simulink model "untitled_H"  (R2013b)
settings: Solver=ode45  StartTime=0.0  StopTime=500  RelTol=1e-3
undefined symbols (not defined in the file): c, delta, kappa, kd, ki, kp, Qs
libraries: simulink x1
settings Model: Creator=Yurii  LastModifiedBy=Yurii

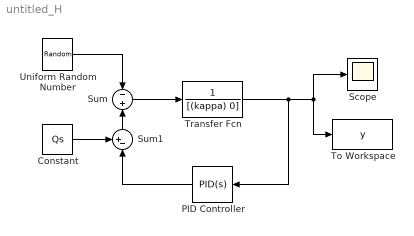
== system untitled_H ==
  Constant : Constant  Value=Qs
  PID Controller : simulink/Continuous/PID Controller  Controller=PID  TimeDomain=Continuous-time  SampleTime=1  IntegratorMethod=Forward Euler  FilterMethod=Forward Euler  Form=Parallel  P=kp  I=ki  D=kd  N=100  InitialConditionSource=internal  InitialConditionForIntegrator=0  InitialConditionForFilter=0  ExternalReset=none  LimitOutput=off  UpperSaturationLimit=inf  LowerSaturationLimit=-inf  LinearizeAsGain=on  AntiWindupMode=none  Kb=1  TrackingMode=off  Kt=1  PParamMin=[]  PParamMax=[]  IParamMin=[]  IParamMax=[]  DParamMin=[]  DParamMax=[]  NParamMin=[]  NParamMax=[]  KbParamMin=[]  KbParamMax=[]  KtParamMin=[]  KtParamMax=[]  POutMin=[]  POutMax=[]  IOutMin=[]  IOutMax=[]  DOutMin=[]  DOutMax=[]  NOutMin=[]  NOutMax=[]  KbOutMin=[]  KbOutMax=[]  KtOutMin=[]  KtOutMax=[]  IntegratorOutMin=[]  IntegratorOutMax=[]  FilterOutMin=[]  FilterOutMax=[]  SumOutMin=[]  SumOutMax=[]  SumI1OutMin=[]  SumI1OutMax=[]  SumI2OutMin=[]  SumI2OutMax=[]  SumI3OutMin=[]  SumI3OutMax=[]  SumDOutMin=[]  SumDOutMax=[]  SaturationOutMin=[]  SaturationOutMax=[]  IntegratorContinuousStateAttributes=''  IntegratorStateMustResolveToSignalObject=off  IntegratorRTWStateStorageClass=Auto  FilterContinuousStateAttributes=''  FilterStateMustResolveToSignalObject=off  FilterRTWStateStorageClass=Auto
  Scope : Scope
  Sum : Sum  Inputs=-|+
  Sum1 : Sum  Inputs=+-|
  To Workspace : ToWorkspace  VariableName=y  SampleTime=-1  SaveFormat=Timeseries
  Transfer Fcn : TransferFcn  Denominator=[(kappa) 0]
  Uniform Random Number : UniformRandomNumber  Minimum=(c-delta)*Qs  Maximum=(c+delta)*Qs  SampleTime=0.1
  wires:
  Uniform Random Number/1 -> Sum/1
  Sum/1 -> Transfer Fcn/1
  Transfer Fcn/1 -> PID Controller/1, To Workspace/1, Scope/1
  Constant/1 -> Sum1/1
  Sum1/1 -> Sum/2
  PID Controller/1 -> Sum1/2
